simulink model "P7"  (R2023b)
settings: Solver=VariableStepAuto  StartTime=0.0  StopTime=10.0  MaxStep=0.001  RelTol=1e-3
values from neighbouring files (symbols this model uses):
  C1 = 100e-9    (= 1e-07)    [ParametrosP7.m]    (also in opamp.m)
  C2 = 100e-9    (= 1e-07)    [ParametrosP7.m]    (also in opamp.m)
  R1 = 5e6    (= 5000000)    [ParametrosP7.m]    (also in opamp.m)
  R2 = 5e6    (= 5000000)    [ParametrosP7.m]    (also in opamp.m)
  R3 = 5e6    (= 5000000)    [ParametrosP7.m]    (also in opamp.m)
libraries: fl_lib x10, nesl_utility x2
settings Model: Creator=aquet  LastModifiedBy=aquet

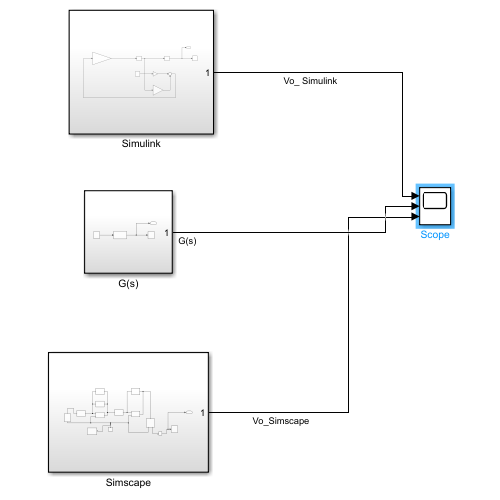
[thumbnail: Simulink's stored preview of the top-level diagram]
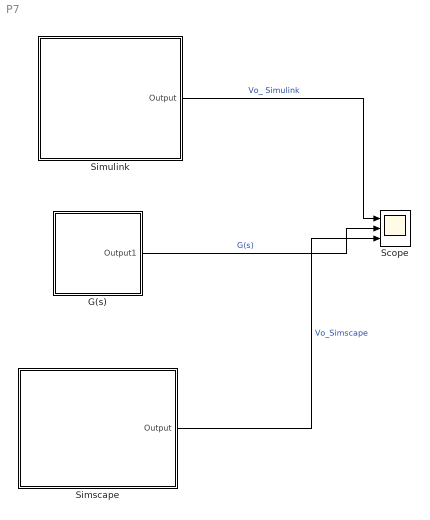
== system P7 ==
  G(s) : Subsystem
  Scope : Scope  NumInputPorts=3
  Simscape : Subsystem
  Simulink : Subsystem
  wires:
  G(s)/1(Output1) -> Scope/2  "G(s)"
  Simulink/1(Output) -> Scope/1  "Vo_ Simulink"
  Simscape/1(Output) -> Scope/3  "Vo_Simscape"

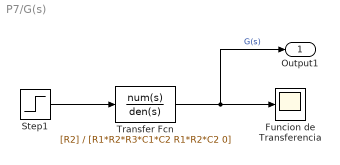
== system P7/G(s) ==
  Funcion de Transferencia : Scope
  Step1 : Step  Time=0  After=5  SampleTime=0
  Transfer Fcn : TransferFcn  Numerator=[R2]  Denominator=[R1*R2*R3*C1*C2 R1*R2*C2 0]
  Output1 : Outport
  wires:
  Step1/1 -> Transfer Fcn/1
  Transfer Fcn/1 -> Output1/1, Funcion de Transferencia/1  "G(s)"

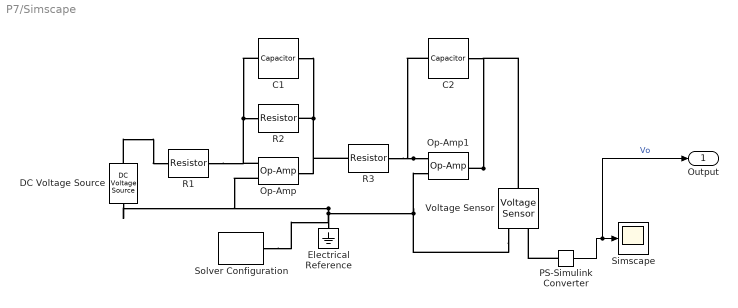
== system P7/Simscape ==
  C1 : fl_lib/Electrical/Electrical Elements/Capacitor  c=100 nF  r=1e-6 Ohm  g=0 1/Ohm  i_specify=off  i_priority=None  i=0 A  i_nominal_specify=off  i_nominal_unit=A  i_nominal_value=1  v_specify=off  v_priority=None  v=0 V  v_nominal_specify=off  v_nominal_unit=V  v_nominal_value=1  vc_specify=off  vc_priority=High  vc=0 V  vc_nominal_specify=off  vc_nominal_unit=V  vc_nominal_value=1
  C2 : fl_lib/Electrical/Electrical Elements/Capacitor  c=100 nF  r=1e-6 Ohm  g=0 1/Ohm  i_specify=off  i_priority=None  i=0 A  i_nominal_specify=off  i_nominal_unit=A  i_nominal_value=1  v_specify=off  v_priority=None  v=0 V  v_nominal_specify=off  v_nominal_unit=V  v_nominal_value=1  vc_specify=off  vc_priority=High  vc=0 V  vc_nominal_specify=off  vc_nominal_unit=V  vc_nominal_value=1
  DC Voltage Source : fl_lib/Electrical/Electrical Sources/DC Voltage Source  v0=5 V
  Electrical Reference : fl_lib/Electrical/Electrical Elements/Electrical Reference
  Op-Amp : fl_lib/Electrical/Electrical Elements/Op-Amp  outI_specify=off  outI_priority=None  outI=0 A  outI_nominal_specify=off  outI_nominal_unit=A  outI_nominal_value=1
  Op-Amp1 : fl_lib/Electrical/Electrical Elements/Op-Amp  outI_specify=off  outI_priority=None  outI=0 A  outI_nominal_specify=off  outI_nominal_unit=A  outI_nominal_value=1
  PS-Simulink Converter : nesl_utility/PS-Simulink Converter  PhysicalDomain=network_engine_domain  SubClassName=ps_output  LeftPortType=input  RightPortType=output  PseudoPeriodic=off  Frequencies=[]  VectorFormat=inherit  Unit=inherit  AffineConversion=off
  R1 : fl_lib/Electrical/Electrical Elements/Resistor  R=5 MOhm  i_specify=off  i_priority=None  i=0 A  i_nominal_specify=off  i_nominal_unit=A  i_nominal_value=1  v_specify=off  v_priority=None  v=0 V  v_nominal_specify=off  v_nominal_unit=V  v_nominal_value=1
  R2 : fl_lib/Electrical/Electrical Elements/Resistor  R=5 MOhm  i_specify=off  i_priority=None  i=0 A  i_nominal_specify=off  i_nominal_unit=A  i_nominal_value=1  v_specify=off  v_priority=None  v=0 V  v_nominal_specify=off  v_nominal_unit=V  v_nominal_value=1
  R3 : fl_lib/Electrical/Electrical Elements/Resistor  R=5 MOhm  i_specify=off  i_priority=None  i=0 A  i_nominal_specify=off  i_nominal_unit=A  i_nominal_value=1  v_specify=off  v_priority=None  v=0 V  v_nominal_specify=off  v_nominal_unit=V  v_nominal_value=1
  Simscape : Scope
  Solver Configuration : nesl_utility/Solver Configuration  PhysicalDomain=network_engine_domain  SubClassName=solver  LeftPortType=input  RightPortType=generic  Tones=[]  Harmonics=[]  SimulateNoise=off  Profile=off  UseLocalSampling=off  EnableSwitchedLinearOptims=on  FrequencyDomain=off  UseCCode=off  RelTol=0.001  AbsTol=0.001  MinStep=1e-09  ToWorkspace=off  RevertToSquareIcSolve=off  NumHomotopyIterations=100  PhasorMode=off  PhasorModeNumHarmonics=1  ConsistencySolver=NEWTON_XTOL_AFTER_FTOL  IndexReductionMethod=DerivativeReplacement  DoDC=off  ResidualTolerance=1e-09  ConsistencyTolSource=GLOBAL  ConsistencyAbsTol=0.001  ConsistencyRelTol=0.001  ConsistencyTolFactor=0.001  UseLocalSolver=off  LocalSolverChoice=NE_BACKWARD_EULER_ADVANCER  ResolveIndetEquations=on  FunctionEvalNumThread=1  LocalSolverSampleTime=0.001  DoFixedCost=off  MaxNonlinIter=3  MaxModeIter=2  ComputeImpulses=off  ImpulseIterations=2  LinearAlgebra=auto  LinearAlgebraNumThread=0  EquationFormulation=NE_TIME_EF  DelaysMemoryBudget=1024  AutomaticFiltering=on  FilteringTimeConstant=0.001  PartitionStorageMethod=AS_NEEDED  PartitionMemoryBudget=1024  PartitionMethod=ROBUST  MultibodyUseLocalSolver=off  MultibodyLocalSolverChoice=ODE1  MultibodyLocalSolverSampleTime=0.001
  Voltage Sensor : fl_lib/Electrical/Electrical Sensors/Voltage Sensor
  Output : Outport
  wires:
  PS-Simulink Converter/1 -> Output/1, Simscape/1  "Vo"
  connections:
  PS-Simulink Converter/LConn1 -- Voltage Sensor/RConn1
  Op-Amp1/RConn1 -- C2/RConn1 -- Voltage Sensor/LConn1
  Op-Amp1/LConn2 -- R3/RConn1 -- C2/LConn1
  Electrical Reference/LConn1 -- Op-Amp/LConn1 -- DC Voltage Source/RConn1 -- Voltage Sensor/RConn2 -- Op-Amp1/LConn1 -- Solver Configuration/RConn1
  R2/LConn1 -- C1/LConn1 -- Op-Amp/LConn2 -- R1/RConn1
  R2/RConn1 -- C1/RConn1 -- R3/LConn1 -- Op-Amp/RConn1
  DC Voltage Source/LConn1 -- R1/LConn1

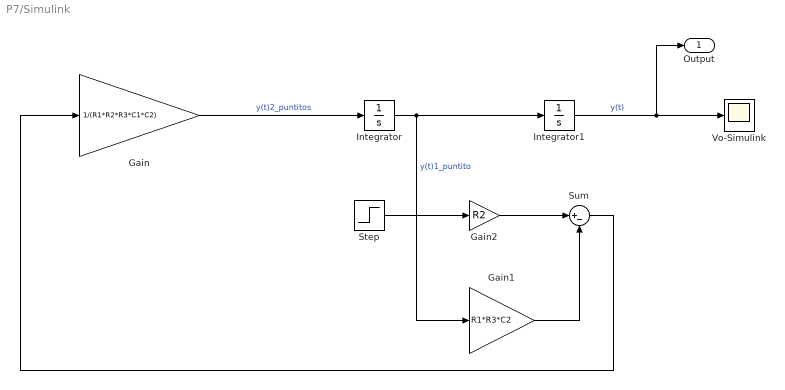
== system P7/Simulink ==
  Gain : Gain  Gain=1/(R1*R2*R3*C1*C2)
  Gain1 : Gain  Gain=R1*R3*C2
  Gain2 : Gain  Gain=R2
  Integrator : Integrator
  Integrator1 : Integrator
  Step : Step  Time=0  After=5  SampleTime=0
  Sum : Sum  Inputs=|+-
  Vo-Simulink : Scope
  Output : Outport
  wires:
  Integrator1/1 -> Output/1, Vo-Simulink/1  "y(t)"
  Gain2/1 -> Sum/1
  Gain1/1 -> Sum/2
  Integrator/1 -> Gain1/1, Integrator1/1  "y(t)1_puntito"
  Sum/1 -> Gain/1
  Gain/1 -> Integrator/1  "y(t)2_puntitos"
  Step/1 -> Gain2/1
